simulink model "sampleModel1593"  (R2023a)
settings: Solver=VariableStepAuto  StartTime=0.0  StopTime=10.0  RelTol=1e-3
libraries: hdlsllib x7, simulink x3
settings Model: Creator=user1  LastModifiedBy=user1

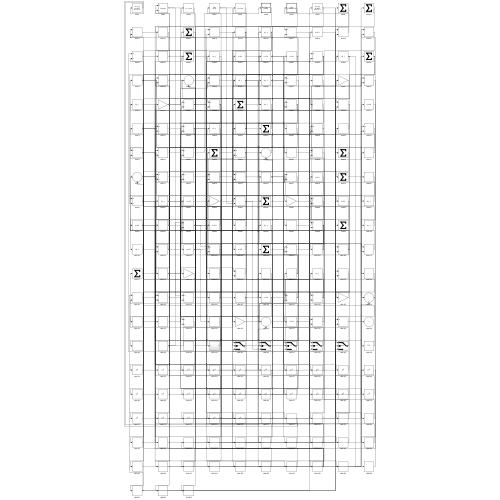
[thumbnail: Simulink's stored preview of the top-level diagram]
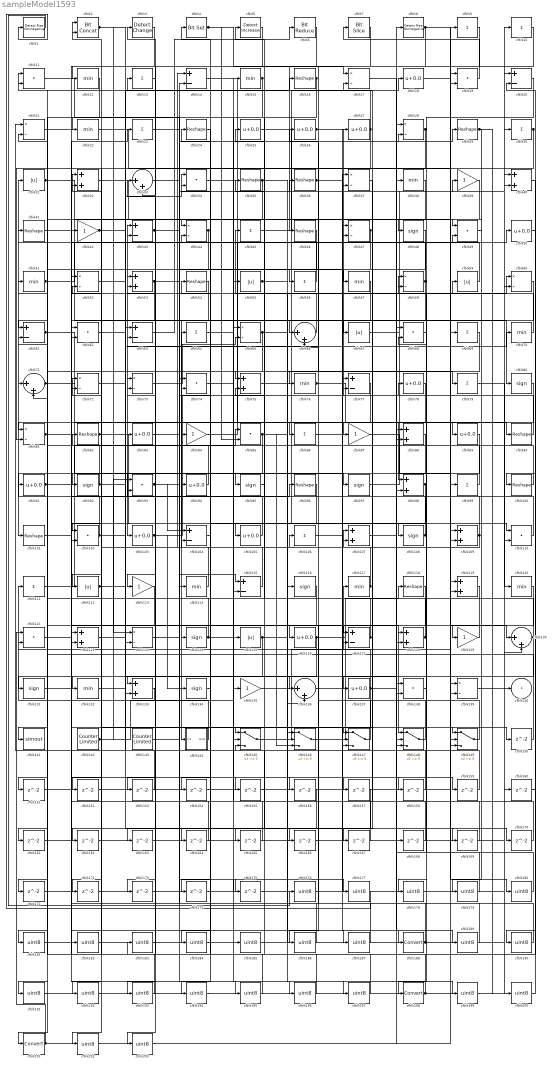
== system sampleModel1593 ==
  cfblk1 : hdlsllib/Logic and Bit Operations/Detect Rise Nonnegative  vinit=0  OutDataTypeStr=boolean
  cfblk{9..10,13,23,30,45,56,64,69,79,86,99,106,111} (14 alike) : Sum  Inputs=+
  cfblk{16,24,29,35..36,41,46,54,82,90,96,100..101,118} (14 alike) : Reshape
  cfblk{11,19,34,49,62,68,74,85,93,102,110,121,138} (13 alike) : DotProduct  OutDataTypeStr=Inherit: Inherit via internal rule
  cfblk{18,25..27,50,78,83,89,91,94,103,105,126,137} (14 alike) : Bias  Bias=0.0  SaturateOnIntegerOverflow=off
  cfblk{14,20,43,61,63,77,104,115,127} (9 alike) : Sum  Inputs=+-
  cfblk{32,40,53,75,88,98,107,109,119,122,128,133} (12 alike) : Sum
  cfblk{48,80,92,95,97,108,116,124,131,134} (10 alike) : Signum
  cfblk{31,55,59,67,112,125} (6 alike) : Abs  SaturateOnIntegerOverflow=off
  cfblk{39,42,84,87,113,129,135} (7 alike) : Gain
  cfblk{12,15,22,38,51,57,70,76,114,117,120,132} (12 alike) : MinMax
  cfblk{17,21,28,37,44,47,52,58,60,65,72..73,81,123,139} (15 alike) : Product  Inputs=*/  RndMeth=Zero  SaturateOnIntegerOverflow=on
  cfblk{33,66,71,130,136} (5 alike) : Sum  Inputs=|++
  cfblk141 : ToWorkspace  VariableName=simout  SaveFormat=Timeseries  SampleTime=-1
  cfblk142 : hdlsllib/Sources/Counter Limited  uplimit=7  tsamp=-1
  cfblk143 : hdlsllib/Sources/Counter Limited  uplimit=7  tsamp=-1
  cfblk144 : Subsystem
      settings: LibrarySourceBlock=|
      | hdlsllib/Ports &
      | Subsystems/Subsystem
  cfblk{145..149} (5 alike) : Switch  SaturateOnIntegerOverflow=off  InputSameDT=off
  cfblk{150..175} (26 alike) : Delay  SampleTime=1
  cfblk{176..187,189..197,199..200,202..203} (25 alike) : DataTypeConversion  OutDataTypeStr=uint8  SaturateOnIntegerOverflow=off  RndMeth=Floor
  cfblk188 : DataTypeConversion  SaturateOnIntegerOverflow=off  RndMeth=Floor
  cfblk198 : DataTypeConversion  SaturateOnIntegerOverflow=off  RndMeth=Floor
  cfblk2 : hdlsllib/Logic and Bit Operations/Bit Concat  numInputs=2
  cfblk201 : DataTypeConversion  SaturateOnIntegerOverflow=off  RndMeth=Floor
  cfblk3 : simulink/Logic and Bit Operations/Detect Change  vinit=0  OutDataTypeStr=boolean
      settings: LibrarySourceBlock=|
      | hdlsllib/Logic and Bit
      | Operations/Detect
      | Change
  cfblk4 : simulink/Logic and Bit Operations/Bit Set  iBit=0
      settings: LibrarySourceBlock=|
      | hdlsllib/Logic and Bit
      | Operations/Bit Set
  cfblk5 : simulink/Logic and Bit Operations/Detect Increase  vinit=0.0  OutDataTypeStr=boolean
      settings: LibrarySourceBlock=|
      | hdlsllib/Logic and Bit
      | Operations/Detect
      | Increase
  cfblk6 : hdlsllib/Logic and Bit Operations/Bit Reduce  mode=AND
  cfblk7 : hdlsllib/Logic and Bit Operations/Bit Slice  lidx=7  ridx=0
  cfblk8 : hdlsllib/Logic and Bit Operations/Detect Rise Nonnegative  vinit=0  OutDataTypeStr=boolean
  cfblk140 : Outport  VectorParamsAs1DForOutWhenUnconnected=off
  wires:
  cfblk75/1 -> cfblk108/1
  cfblk44/1 -> cfblk161/1, cfblk184/1
  cfblk20/1 -> cfblk198/1
  cfblk2/1 -> cfblk123/1, cfblk107/2
  cfblk148/1 -> cfblk14/1
  cfblk98/1 -> cfblk148/3, cfblk167/1, cfblk194/1
  cfblk61/1 -> cfblk89/1, cfblk156/1
  cfblk65/1 -> cfblk112/1, cfblk199/1
  cfblk28/1 -> cfblk145/1, cfblk162/1, cfblk191/1
  cfblk94/1 -> cfblk43/1
  cfblk102/1 -> cfblk31/1, cfblk169/1
  cfblk90/1 -> cfblk27/1
  cfblk108/1 -> cfblk71/1, cfblk44/2
  cfblk63/1 -> cfblk6/1
  cfblk29/1 -> cfblk129/1, cfblk200/1
  cfblk57/1 -> cfblk144/1(In1)
  cfblk134/1 -> cfblk21/1
  cfblk124/1 -> cfblk125/1, cfblk53/1
  cfblk12/1 -> cfblk22/1
  cfblk10/1 -> cfblk113/1
  cfblk45/1 -> cfblk18/1
  cfblk25/1 -> cfblk87/1
  cfblk15/1 -> cfblk61/1, cfblk115/2
  cfblk59/1 -> cfblk47/1
  cfblk9/1 -> cfblk133/1
  cfblk6/1 -> cfblk46/1
  cfblk14/1 -> cfblk86/1
  cfblk114/1 -> cfblk64/1
  cfblk66/1 -> cfblk45/1
  cfblk32/1 -> cfblk135/1
  cfblk105/1 -> cfblk73/1
  cfblk11/1 -> cfblk114/1
  cfblk129/1 -> cfblk126/1
  cfblk55/1 -> cfblk5/1, cfblk147/2
  cfblk8/1 -> cfblk56/1, cfblk180/1
  cfblk7/1 -> cfblk66/1
  cfblk97/1 -> cfblk10/1
  cfblk82/1 -> cfblk105/1, cfblk138/2
  cfblk136/1 -> cfblk37/1
  cfblk143/1 -> cfblk14/2
  cfblk84/1 -> cfblk8/1
  cfblk24/1 -> cfblk124/1
  cfblk67/1 -> cfblk30/1
  cfblk103/1 -> cfblk77/1, cfblk134/1
  cfblk58/1 -> cfblk123/2, cfblk13/1
  cfblk133/1 -> cfblk111/1
  cfblk48/1 -> cfblk133/2
  cfblk16/1 -> cfblk95/1, cfblk145/2
  cfblk146/1 -> cfblk118/1
  cfblk149/1 -> cfblk94/1
  cfblk80/1 -> cfblk98/1
  cfblk34/1 -> cfblk99/1
  cfblk78/1 -> cfblk131/1
  cfblk128/1 -> cfblk61/2, cfblk91/1
  cfblk26/1 -> cfblk90/1, cfblk48/1
  cfblk95/1 -> cfblk25/1
  cfblk125/1 -> cfblk60/1, cfblk171/1
  cfblk127/1 -> cfblk32/1, cfblk107/1
  cfblk50/1 -> cfblk100/1
  cfblk52/1 -> cfblk83/1
  cfblk111/1 -> cfblk85/1
  cfblk145/1 -> cfblk109/1
  cfblk71/1 -> cfblk97/1, cfblk49/2, cfblk53/2
  cfblk31/1 -> cfblk80/1, cfblk168/1
  cfblk3/1 -> cfblk62/2
  cfblk46/1 -> cfblk132/1
  cfblk35/1 -> cfblk79/1, cfblk110/2, cfblk202/1
  cfblk135/1 -> cfblk117/1
  cfblk30/1 -> cfblk75/1, cfblk49/1
  cfblk73/1 -> cfblk65/2
  cfblk99/1 -> cfblk2/1
  cfblk120/1 -> cfblk148/1
  cfblk87/1 -> cfblk139/2
  cfblk132/1 -> cfblk70/1
  cfblk37/1 -> cfblk147/1
  cfblk43/1 -> cfblk3/1, cfblk29/1, cfblk175/1
  cfblk137/1 -> cfblk51/1, cfblk172/1, cfblk189/1
  cfblk106/1 -> cfblk188/1
  cfblk36/1 -> cfblk47/2, cfblk110/1
  cfblk60/1 -> cfblk102/1
  cfblk91/1 -> cfblk148/2, cfblk157/1
  cfblk53/1 -> cfblk128/1, cfblk72/2, cfblk170/1
  cfblk115/1 -> cfblk24/1
  cfblk19/1 -> cfblk7/1
  cfblk88/1 -> cfblk101/1
  cfblk123/1 -> cfblk36/1
  cfblk119/1 -> cfblk201/1
  cfblk109/1 -> cfblk2/2, cfblk58/2, cfblk104/2
  cfblk47/1 -> cfblk76/1, cfblk153/1
  cfblk100/1 -> cfblk21/2
  cfblk64/1 -> cfblk39/1
  cfblk139/1 -> cfblk60/2
  cfblk117/1 -> cfblk84/1, cfblk52/2
  cfblk4/1 -> cfblk17/1, cfblk85/2
  cfblk122/1 -> cfblk16/1
  cfblk92/1 -> cfblk11/1, cfblk150/1, cfblk152/1
  cfblk113/1 -> cfblk122/2
  cfblk56/1 -> cfblk41/1
  cfblk107/1 -> cfblk50/1
  cfblk142/1 -> cfblk55/1, cfblk93/1
  cfblk130/1 -> cfblk137/1, cfblk75/2
  cfblk51/1 -> cfblk67/1, cfblk15/1, cfblk23/1
  cfblk76/1 -> cfblk128/2, cfblk159/1
  cfblk147/1 -> cfblk63/2
  cfblk22/1 -> cfblk69/1
  cfblk85/1 -> cfblk146/1, cfblk146/3, cfblk173/1
  cfblk69/1 -> cfblk81/1
  cfblk17/1 -> cfblk88/1
  cfblk23/1 -> cfblk57/1
  cfblk27/1 -> cfblk141/1, cfblk81/2, cfblk11/2
  cfblk72/1 -> cfblk59/1
  cfblk42/1 -> cfblk34/1, cfblk44/1
  cfblk138/1 -> cfblk78/1
  cfblk54/1 -> cfblk92/1
  cfblk144/1(Out1) -> cfblk73/2
  cfblk112/1 -> cfblk58/1, cfblk166/1
  cfblk79/1 -> cfblk120/1
  cfblk70/1 -> cfblk35/1
  cfblk121/1 -> cfblk96/1
  cfblk126/1 -> cfblk28/1, cfblk174/1
  cfblk89/1 -> cfblk103/1
  cfblk83/1 -> cfblk28/2
  cfblk81/1 -> cfblk127/1, cfblk109/2
  cfblk5/1 -> cfblk12/1
  cfblk62/1 -> cfblk136/1
  cfblk110/1 -> cfblk72/1
  cfblk101/1 -> cfblk149/1
  cfblk18/1 -> cfblk130/1
  cfblk93/1 -> cfblk115/1, cfblk104/1, cfblk77/2
  cfblk150/1 -> cfblk71/2
  cfblk39/1 -> cfblk151/1
  cfblk151/1 -> cfblk102/2
  cfblk152/1 -> cfblk136/2
  cfblk153/1 -> cfblk63/1
  cfblk77/1 -> cfblk154/1
  cfblk21/1 -> cfblk155/1
  cfblk155/1 -> cfblk139/1
  cfblk86/1 -> cfblk158/1
  cfblk158/1 -> cfblk43/2
  cfblk159/1 -> cfblk34/2
  cfblk162/1 -> cfblk127/2
  cfblk13/1 -> cfblk163/1
  cfblk163/1 -> cfblk37/2
  cfblk104/1 -> cfblk164/1
  cfblk164/1 -> cfblk62/1
  cfblk96/1 -> cfblk165/1
  cfblk165/1 -> cfblk65/1
  cfblk166/1 -> cfblk130/2
  cfblk167/1 -> cfblk66/2
  cfblk168/1 -> cfblk32/2
  cfblk169/1 -> cfblk17/2
  cfblk170/1 -> cfblk149/2
  cfblk171/1 -> cfblk147/3
  cfblk172/1 -> cfblk146/2
  cfblk173/1 -> cfblk149/3
  cfblk175/1 -> cfblk88/2
  cfblk1/1 -> cfblk176/1
  cfblk176/1 -> cfblk26/1
  cfblk174/1 -> cfblk177/1
  cfblk177/1 -> cfblk1/1
  cfblk68/1 -> cfblk178/1
  cfblk178/1 -> cfblk140/1
  cfblk49/1 -> cfblk179/1
  cfblk179/1 -> cfblk68/1
  cfblk180/1 -> cfblk68/2
  cfblk116/1 -> cfblk181/1
  cfblk181/1 -> cfblk42/1
  cfblk131/1 -> cfblk182/1
  cfblk182/1 -> cfblk116/1
  cfblk160/1 -> cfblk183/1
  cfblk183/1 -> cfblk19/1
  cfblk184/1 -> cfblk160/1
  cfblk74/1 -> cfblk185/1
  cfblk185/1 -> cfblk19/2
  cfblk118/1 -> cfblk186/1
  cfblk186/1 -> cfblk74/1
  cfblk161/1 -> cfblk187/1
  cfblk187/1 -> cfblk74/2
  cfblk188/1 -> cfblk93/2, cfblk122/1
  cfblk189/1 -> cfblk106/1
  cfblk40/1 -> cfblk190/1
  cfblk190/1 -> cfblk138/1
  cfblk191/1 -> cfblk40/1
  cfblk156/1 -> cfblk192/1
  cfblk192/1 -> cfblk40/2
  cfblk38/1 -> cfblk193/1
  cfblk193/1 -> cfblk82/1
  cfblk194/1 -> cfblk38/1
  cfblk33/1 -> cfblk195/1
  cfblk195/1 -> cfblk4/1
  cfblk41/1 -> cfblk196/1
  cfblk196/1 -> cfblk33/1
  cfblk154/1 -> cfblk197/1
  cfblk197/1 -> cfblk33/2
  cfblk198/1 -> cfblk145/3, cfblk121/2, cfblk52/1, cfblk54/1
  cfblk199/1 -> cfblk20/1
  cfblk200/1 -> cfblk20/2
  cfblk201/1 -> cfblk98/2, cfblk121/1, cfblk9/1
  cfblk202/1 -> cfblk119/1
  cfblk157/1 -> cfblk203/1
  cfblk203/1 -> cfblk119/2

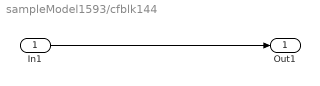
== system sampleModel1593/cfblk144 ==
  In1 : Inport
  Out1 : Outport
  wires:
  In1/1 -> Out1/1
